simulink model "HMI_SimulinkSetup"  (R2024b)
settings: Solver=FixedStepDiscrete  StartTime=0.0  StopTime=inf  FixedStep=0.001  RelTol=1e-3
libraries: simulink x1, dspstat3 x1, dspnetwork x1
settings Model: Creator=mehme  LastModifiedBy=mehme

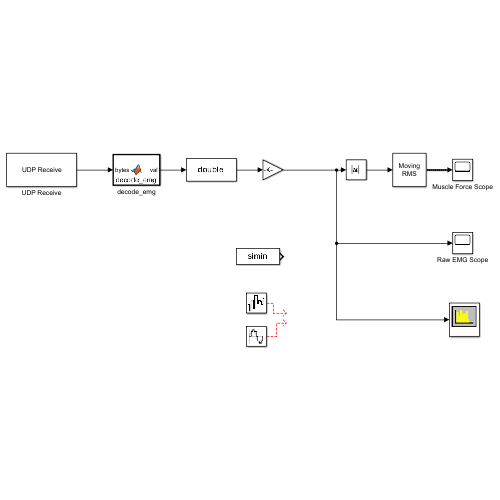
[thumbnail: Simulink's stored preview of the top-level diagram]
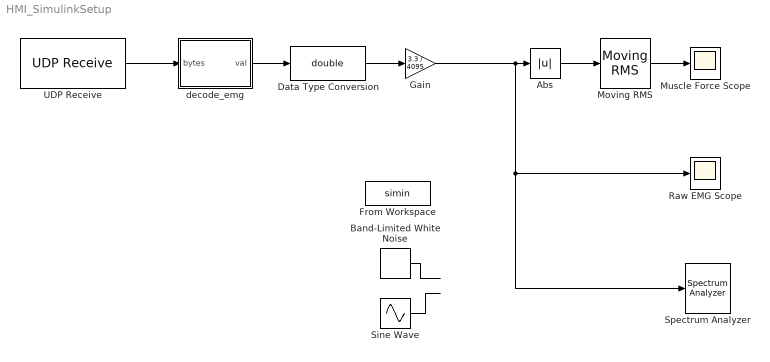
== system HMI_SimulinkSetup ==
  Abs : Abs  SaturateOnIntegerOverflow=off
  Band-Limited White Noise : simulink/Sources/Band-Limited White Noise  Cov=0.0001  Ts=0.001  seed=[23341]
  Data Type Conversion : DataTypeConversion  OutDataTypeStr=double  SaturateOnIntegerOverflow=off  RndMeth=Floor
  From Workspace : FromWorkspace  VariableName=simin  SampleTime=0.001  Interpolate=off  OutputAfterFinalValue=Setting to zero
  Gain : Gain  Gain=3.3 / 4095
  Moving RMS : dspstat3/Moving RMS  Method=Sliding window  ForgettingFactorPort=off  SpecifyWindowLength=on  WindowLength=200  OverlapLength=199  AllowArbitraryInputLength=on  ForgettingFactor=0.9  SimulateUsing=Interpreted execution
  Muscle Force Scope : Scope
  Raw EMG Scope : Scope
  Sine Wave : Sin  Frequency=50  SampleTime=0.001
  Spectrum Analyzer : SpectrumAnalyzer  WindowPosition=[633.000000,100.000000,800.000000,500.000000,]  ScopeFrameLocation=window  WindowInvariantSamplesPerUpdate=on  YLimits=[-27.409377191623378,24.414948617021263]
  UDP Receive : dspnetwork/UDP Receive  localURL='0.0.0.0'  localPort=25000  remoteURL='0.0.0.0'  remotePort=-1  recvBufferSize=8192  dims=255  signalDatatype=uint8  isComplex=off  isVarSize=on  showBlockingTime=off  blockingTime=0  sampletime=1  blockPlatform=[]
      settings: LibrarySourceBlock=dspsrcs4/UDP Receive
  decode_emg : MATLAB Function  TreatAsAtomicUnit=on
  wires:
  Abs/1 -> Moving RMS/1
  Moving RMS/1 -> Muscle Force Scope/1
  Band-Limited White Noise/1 -> ?
  Sine Wave/1 -> ?
  decode_emg/1(val) -> Data Type Conversion/1
  Gain/1 -> Raw EMG Scope/1, Spectrum Analyzer/1, Abs/1
  Data Type Conversion/1 -> Gain/1
  UDP Receive/1 -> decode_emg/1(bytes)

== matlab function HMI_SimulinkSetup/decode_emg ==
  data: bytes input; val output
function val = decode_emg(bytes)
    % Input 'bytes' is a vector of 2 numbers (uint8)
    % We assume STM32 sends [LowByte, HighByte]
    
    % Combine them: Low + (High * 256)
    %The STM32 sends a 16-bit integer split into two 8-bit pieces. This puts them back together.
    val = double(bytes(1)) + (double(bytes(2)) * 256);
end
